simulink model "Model_DC_MG"  (R2024b)
settings: Solver=ode23tb  StartTime=0.0  StopTime=3  MaxStep=1e-2  RelTol=1e-3
InitFcn:
  | Main_DC_MG
undefined symbols (not defined in the file or in its folder): DiscIntNeverNeededParam, Ion, Lithium, R_Load_DC, sigbuilder_block, Ts_Control, Ts_Power, V2G, Vnom_DC
libraries: spsSeriesRLCBranchLib x9, spsMeanLib x9, simulink x8, spsBreakerLib x7, spsCurrentMeasurementLib x5, spsVoltageMeasurementLib x4, spsIGBTDiodeLib x2, spsFourierLib x2, spsPVArrayLib x1, spsBatteryLib x1, spsDiodeLib x1, spsIGBTLib x1
settings Model: Creator=Leony  LastModifiedBy=ASUS
settings SolverCC: ZeroCrossAlgorithm=Adaptive  AlgebraicLoopSolver=TrustRegion  SolverResetMethod=Robust
settings DataIOCC: LimitDataPoints=on  SaveFormat=Array  ReturnWorkspaceOutputs=off
settings OptimizationCC: LifeSpan=inf
settings DebuggingCC: AlgebraicLoopMsg=none  UnderspecifiedInitializationDetection=Classic  MergeDetectMultiDrivingBlocksExec=none  IgnoredZcDiagnostic=none  SolverPrmCheckMsg=warning  UnconnectedInputMsg=warning  UnconnectedOutputMsg=warning  UnconnectedLineMsg=warning  AllowSymbolicDim=off  SFUnexpectedBacktrackingDiag=warning  SFNoUnconditionalDefaultTransitionDiag=warning  SFExecutionAtInitializationDiag=none  ArithmeticOperatorsInVariantConditions=warning
settings HardwareCC: ProdBitPerPointer=32  ProdBitPerSizeT=32  ProdBitPerPtrDiffT=32  ProdLargestAtomicFloat=None  ProdIntDivRoundTo=Undefined  ProdEndianess=Unspecified  ProdWordSize=32  ProdHWDeviceType=32-bit Generic
settings ModelReferenceCC: EnableRefExpFcnMdlSchedulingChecks=on  PropagateSignalLabelsOutOfModel=off
settings SFSimCC: SimUseLocalCustomCode=off  CustomCodeUndefinedFunction=UseInterfaceOnly
settings RTWCC: RTWUseLocalCustomCode=off  GPUComputeCapability=3.5
settings CodeAppCC: StateflowObjectComments=on
settings GRTTargetCC: TargetLangStandard=C89/C90 (ANSI)
settings ConfigComp: CovMetricSettings=dw  CovSaveCumulativeToWorkspaceVar=on  CovSaveSingleToWorkspaceVar=on  CovExternalEMLEnable=off
settings SimscapeCC: SimscapeNormalizeSystem=off

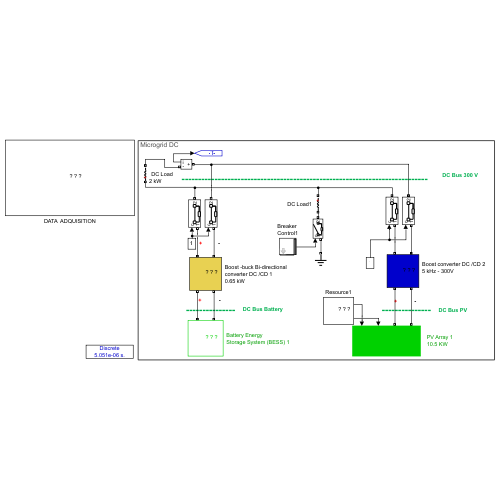
[thumbnail: Simulink's stored preview of the top-level diagram]
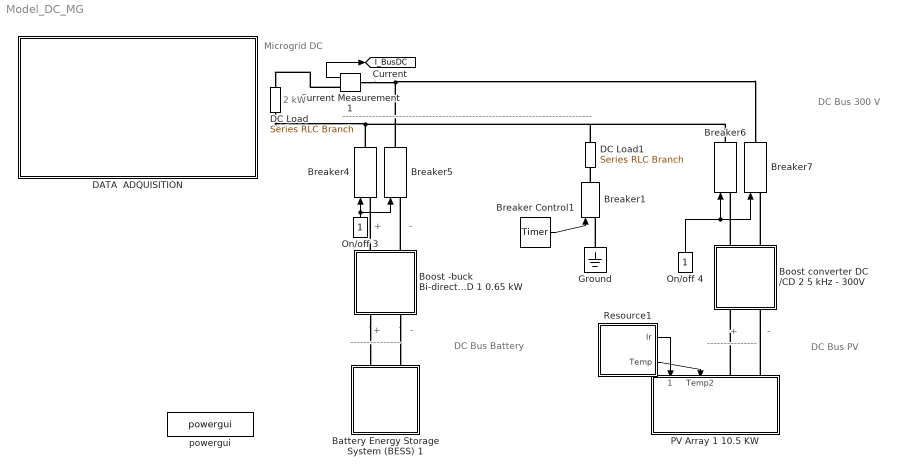
== system Model_DC_MG ==
  note: ---------------------------------------------------------------------------
  note: DC Bus 300 V
  note: 2 kW
  note: DC Bus Battery
  note: +
  note: -
  note: +
  note: ---------------
  note: -
  note: ---------------
  note: +
  note: -
  note: DC Bus PV
  note: Microgrid DC
  "  PV Array 1 10.5 KW" : Subsystem
      mask Display: image(imread('Icons\PV.png'));
  Battery Energy Storage System (BESS) 1 : Subsystem
      mask Display: image('Icons\Battery Energy Storage System (BESS).png');
  Boost -buck Bi-directional converter DC /CD 1 0.65 kW : Subsystem
      mask Display: image(imread('Icons\DC_DC_Converter.jpg'));
  "Boost converter DC /CD 2 5 kHz - 300V " : Subsystem
      mask Display: image(imread('Icons\DC_DC_Converter.jpg'));
  Breaker Control1 : powerlib_extras/Control  Blocks/Timer  t=[0 2 2.2]  e=[0 1 0]
  Breaker1 : spsBreakerLib/Breaker  InitialState=0  SwitchingTimes="[1/60  5/60]"  External=on  BreakerResistance=0.01  SnubberResistance=1e6  SnubberCapacitance=inf  Measurements=None  MoreParameters=on  NoBreakLoop=off
  Breaker{4..7} (4 alike) : spsBreakerLib/Breaker  InitialState=1  SwitchingTimes="[1/60  5/60]"  External=on  BreakerResistance=0.01  SnubberResistance=1e6  SnubberCapacitance=inf  Measurements=None  MoreParameters=on  NoBreakLoop=off
  Current Measurement1 : spsCurrentMeasurementLib/Current Measurement  PhasorSimulation=off  OutputType=Complex  PSBequivalent=0
  DATA  ADQUISITION : Subsystem
      mask Display: image('Icons\SCADA.png');
  DC Load : spsSeriesRLCBranchLib/Series RLC Branch  LConnTagsString=__new0  RConnTagsString=__new0  BranchType=R  Resistance=R_Load_DC  Inductance=1e-3  SetiL0=off  InitialCurrent=0  Capacitance=1e-6  Setx0=off  InitialVoltage=0  Measurements=None
  DC Load1 : spsSeriesRLCBranchLib/Series RLC Branch  LConnTagsString=__new0  RConnTagsString=__new0  BranchType=R  Resistance=0.001  Inductance=1e-3  SetiL0=off  InitialCurrent=0  Capacitance=1e-6  Setx0=off  InitialVoltage=0  Measurements=None
  Ground : spsGroundLib/Ground  LConnTagsString=a
  On/off 3 : Constant
  On/off 4 : Constant
  Resource1 : Subsystem
      mask Display: image(imread('Icons\R_Sol.jpg'));
  powergui : spspowerguiLib/powergui  Priority=1  SimulationMode=Discrete  SampleTime=Ts_Power  frequency=60  Iterations=50  frequencyindice=0  Pbase=100e6  ErrMax=1e-4  UnitsV=kV  UnitsW=MW  buscounter=0  FunctionMessages=off  echomessages=off  EnableUseOfTLC=off  CurrentSourceSwitches=off  DisableSnubberDevices=off  DisableRonSwitches=off  DisableVfSwitches=off  DisplayEquations=off  AutomaticDiscreteSolvers=off  SolverType=Tustin  Interpol=off  ExternalGateDelay=off  methode=off  Ts=0  x0status=blocks  SPID=off  SwTol=0  HookPort=off  NonlinearTolerance=1e-4  nMaxIteration=100  ContinueOnMaxIteration=off  RestoreLinks=warning  ResistiveCurrentMeasurement=off  Frange=[0:2:500]  Ylog=off  Xlog=on  ShowGrid=off  save=off  variable=ZData  structure=0  ZoomFFT=off  StartTime=0.0  cycles=1  DisplayStyle=1  fundamental=60  FreqAxis=off  MaxFrequency=1000  frequencyindicesteady=1  RmsSteady=1  display=off
  tag scope: I_BusDC=global
  wires:
  On/off 3/1 -> Breaker5/1, Breaker4/1
  Resource1/1(Ir) -> "  PV Array 1 10.5 KW"/1(Radiación)
  Resource1/2("Temp ") -> "  PV Array 1 10.5 KW"/2(Temp2)
  Current Measurement1/1 -> [I_BusDC]
  On/off 4/1 -> Breaker7/1, Breaker6/1
  Breaker Control1/1 -> Breaker1/1
  connections:
  Breaker5/RConn1 -- Current Measurement1/LConn1 -- Breaker7/RConn1
  Breaker4/RConn1 -- DC Load1/LConn1 -- Breaker6/RConn1 -- DC Load/LConn1
  Boost -buck Bi-directional converter DC /CD 1 0.65 kW/LConn1 -- Battery Energy Storage System (BESS) 1/LConn1
  Boost -buck Bi-directional converter DC /CD 1 0.65 kW/LConn2 -- Battery Energy Storage System (BESS) 1/LConn2
  Boost -buck Bi-directional converter DC /CD 1 0.65 kW/RConn1 -- Breaker4/LConn1
  Boost -buck Bi-directional converter DC /CD 1 0.65 kW/RConn2 -- Breaker5/LConn1
  "Boost converter DC /CD 2 5 kHz - 300V "/LConn1 -- Breaker6/LConn1
  "Boost converter DC /CD 2 5 kHz - 300V "/LConn2 -- Breaker7/LConn1
  "  PV Array 1 10.5 KW"/LConn2 -- "Boost converter DC /CD 2 5 kHz - 300V "/RConn2
  "  PV Array 1 10.5 KW"/LConn1 -- "Boost converter DC /CD 2 5 kHz - 300V "/RConn1
  Current Measurement1/RConn1 -- DC Load/RConn1
  Breaker1/RConn1 -- DC Load1/RConn1
  Ground/LConn1 -- Breaker1/LConn1

== system Model_DC_MG/  PV Array 1 10.5 KW ==
  note: DC Bus
  note: 10.5 - kW  PV Array
      | 42 * SunTech STP - 250S-20 /Wd  (Nser=6 Npar=7)
  Radiación : Inport
  Temp2 : Inport  Port=2
  PV Array : spsPVArrayLib/PV Array  Npar=7  Nser=6  PlotType=array @ 1000 W/m2 & specified temperatures  S_vec="[ 1000  250 ]"  Temp_C_vec="[0 25 50  ]"  ModuleName=User-defined  PlotWhenSelected=off  Pm=250.205  Ncell=96  Voc=37.4  Isc=8.63  Vm=30.7  Im=8.15  beta_Voc_pc=-0.34  alpha_Isc_pc=0.050  beta_Voc=-0.12716  alpha_Isc=0.004315  IL=8.6686  I0=1.3965e-10  nI=0.6105  Rsh=311.9016  Rs=0.26776  RobustModel=off  RobustCellTemperature=313.3991  BAL=on  Tc=Tc  Tfilter=5e-5
  + : PMIOPort  Tag=PMCPort  Side=Left
  - : PMIOPort  Tag=PMCPort  Port=2  Side=Left
  tag scope: m_PV=global
  wires:
  Temp2/1 -> PV Array/2
  Radiación/1 -> PV Array/1
  PV Array/1 -> [m_PV]
  connections:
  PV Array/RConn1 -- +/RConn1
  PV Array/RConn2 -- -/RConn1

== system Model_DC_MG/Battery Energy Storage System (BESS) 1 ==
  Battery1 : spsBatteryLib/Battery  BatType=Lithium-Ion  NomV=120  NomQ=800  SOC=80  Batt_Tr=3  PresetModel=on  MaxQ=800  MinV=90  FullV=139.6785  Dis_rate=347.8261  R=0.0015  Normal_OP=723.4783  expZone="[129.6463      39.30435]"
      settings: LibrarySourceBlock=electricdrivelib/Extra Sources/Battery
  + B1 : PMIOPort  Side=Left
  - B1 : PMIOPort  Port=2  Side=Left
  connections:
  Battery1/LConn2 -- - B1/RConn1
  Battery1/LConn1 -- + B1/RConn1

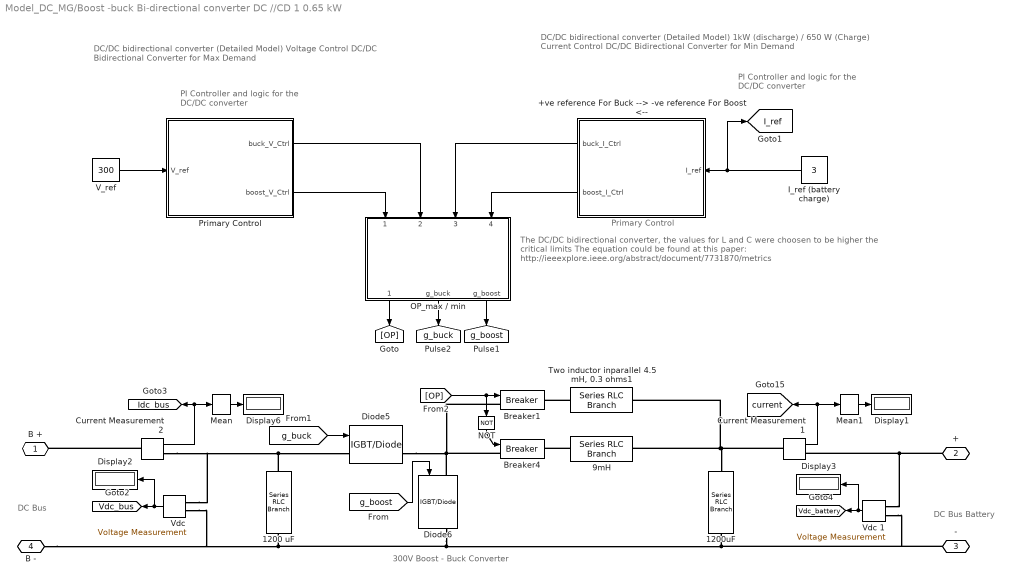
== system Model_DC_MG/Boost -buck Bi-directional converter DC //CD 1 0.65 kW ==
  note: Primary Control
  note: DC Bus
  note: DC Bus Battery
  note: PI Controller and logic for
      | the DC/DC converter
  note: DC/DC bidirectional converter (Detailed Model)
      | Voltage Control DC/DC Bidirectional Converter for Max Demand
  note: 300V
      | Boost - Buck Converter
  note: PI Controller and logic for
      | the DC/DC converter
  note: DC/DC bidirectional converter (Detailed Model)
      | 1kW (discharge) / 650 W (Charge)
      | Current Control DC/DC Bidirectional Converter for Min Demand
  note: The DC/DC bidirectional converter, the values for L and C were choosen to be higher the critical limits The equation could be found at this paper:
      | http://ieeexplore.ieee.org/abstract/document/7731870/metrics
  +ve reference For Buck --> -ve reference For Boost <-- : Subsystem
      mask Display: image('Icons\FPGA.png');
  1200 uF : spsSeriesRLCBranchLib/Series RLC Branch  LConnTagsString=__new0  RConnTagsString=__new0  BranchType=RC  Resistance=0.1  Inductance=3e-3  SetiL0=off  InitialCurrent=0  Capacitance=1200e-6  Setx0=off  InitialVoltage=150  Measurements=None
  1200uF : spsSeriesRLCBranchLib/Series RLC Branch  LConnTagsString=__new0  RConnTagsString=__new0  BranchType=C  Resistance=1  Inductance=3e-3  SetiL0=off  InitialCurrent=0  Capacitance=1200e-6  Setx0=off  InitialVoltage=130  Measurements=None
  9mH : spsSeriesRLCBranchLib/Series RLC Branch  LConnTagsString=__new0  RConnTagsString=__new0  BranchType=L  Resistance=1  Inductance=9e-3  SetiL0=off  InitialCurrent=0  Capacitance=1e-6  Setx0=off  InitialVoltage=0  Measurements=None
  Breaker1 : spsBreakerLib/Breaker  InitialState=0  SwitchingTimes="[1/60  5/60]"  External=on  BreakerResistance=0.0001  SnubberResistance=1e6  SnubberCapacitance=inf  Measurements=None  MoreParameters=on  NoBreakLoop=off
  Breaker4 : spsBreakerLib/Breaker  InitialState=0  SwitchingTimes="[1/60  5/60]"  External=on  BreakerResistance=0.0001  SnubberResistance=1e6  SnubberCapacitance=inf  Measurements=None  MoreParameters=on  NoBreakLoop=off
  Current Measurement1 : spsCurrentMeasurementLib/Current Measurement  PhasorSimulation=off  OutputType=Complex  PSBequivalent=0
  Current Measurement2 : spsCurrentMeasurementLib/Current Measurement  PhasorSimulation=off  OutputType=Complex  PSBequivalent=0
  Diode5 : spsIGBTDiodeLib/IGBT//Diode  Ron=1e-3  Rs=1e5  Cs=inf  Measurements=on
  Diode6 : spsIGBTDiodeLib/IGBT//Diode  Ron=1e-3  Rs=1e5  Cs=inf  Measurements=on
  Display{1..3,6} (4 alike) : Display
  I_ref (battery charge) : Constant  Value=3
  Mean : spsMeanLib/Mean  Freq=10  Vinit=0  Ts=0
  Mean1 : spsMeanLib/Mean  Freq=10  Vinit=0  Ts=0
  NOT : Logic  Operator=NOT  IconShape=distinctive  AllPortsSameDT=off  OutDataTypeStr=boolean
  OP_max / min : Subsystem
  Primary Control : Subsystem
      mask Display: image('Icons\FPGA.png');
  "Two inductor inparallel 4.5 mH, 0.3 ohms1" : spsSeriesRLCBranchLib/Series RLC Branch  LConnTagsString=__new0  RConnTagsString=__new0  BranchType=RL  Resistance=.25  Inductance=4.5e-3  SetiL0=off  InitialCurrent=0  Capacitance=1e-6  Setx0=off  InitialVoltage=0  Measurements=None
  V_ref : Constant  Value=300
  "Vdc " : spsVoltageMeasurementLib/Voltage Measurement  Tag=PoWeRsYsTeMmEaSuReMeNt  PhasorSimulation=off  OutputType=Magnitude  PSBequivalent=0
  Vdc 1 : spsVoltageMeasurementLib/Voltage Measurement  Tag=PoWeRsYsTeMmEaSuReMeNt  PhasorSimulation=off  OutputType=Magnitude  PSBequivalent=0
  B + : PMIOPort  Side=Right
  + : PMIOPort  Port=2  Side=Left
  - : PMIOPort  Port=3  Side=Left
  B - : PMIOPort  Port=4  Side=Right
  tag scope: I_ref=global, Idc_bus=global, Vdc_battery=global, Vdc_bus=global, current=global, g_boost=global, g_buck=global
  wires:
  "Vdc "/1 -> Display2/1, [Vdc_bus]
  Vdc 1/1 -> Display3/1, [Vdc_battery]
  Current Measurement2/1 -> Mean/1, [Idc_bus]
  [g_boost] -> Diode6/1
  [g_buck] -> Diode5/1
  Mean/1 -> Display6/1
  Current Measurement1/1 -> [current], Mean1/1
  Mean1/1 -> Display1/1
  V_ref/1 -> Primary Control/1(V_ref)
  OP_max / min/1(Op_Max / Min) -> [OP]
  [OP] -> NOT/1, Breaker1/1
  NOT/1 -> Breaker4/1
  I_ref (battery charge)/1 -> [I_ref], +ve reference For Buck --> -ve reference For Boost <--/1(I_ref)
  +ve reference For Buck --> -ve reference For Boost <--/1(buck_I_Ctrl) -> OP_max / min/3(buck_I_Ctrl)
  +ve reference For Buck --> -ve reference For Boost <--/2(boost_I_Ctrl) -> OP_max / min/4(boost_I_Ctrll)
  OP_max / min/2(g_buck) -> [g_buck]
  OP_max / min/3(g_boost) -> [g_boost]
  Primary Control/1(buck_V_Ctrl) -> OP_max / min/2(buck_V_Ctrl)
  Primary Control/2(boost_V_Ctrl) -> OP_max / min/1(boost_V_Ctrll)
  connections:
  +/RConn1 -- Vdc 1/LConn1 -- Current Measurement1/RConn1
  Diode5/RConn1 -- Breaker1/LConn1 -- Breaker4/LConn1 -- Diode6/LConn1
  1200 uF/LConn1 -- "Vdc "/LConn1 -- Current Measurement2/RConn1 -- Diode5/LConn1
  Diode6/RConn1 -- "Vdc "/LConn2 -- B -/RConn1 -- 1200 uF/RConn1 -- Vdc 1/LConn2 -- -/RConn1 -- 1200uF/RConn1
  Current Measurement2/LConn1 -- B +/RConn1
  "Two inductor inparallel 4.5 mH, 0.3 ohms1"/LConn1 -- Breaker1/RConn1
  Current Measurement1/LConn1 -- 1200uF/LConn1 -- 9mH/RConn1 -- "Two inductor inparallel 4.5 mH, 0.3 ohms1"/RConn1
  9mH/LConn1 -- Breaker4/RConn1

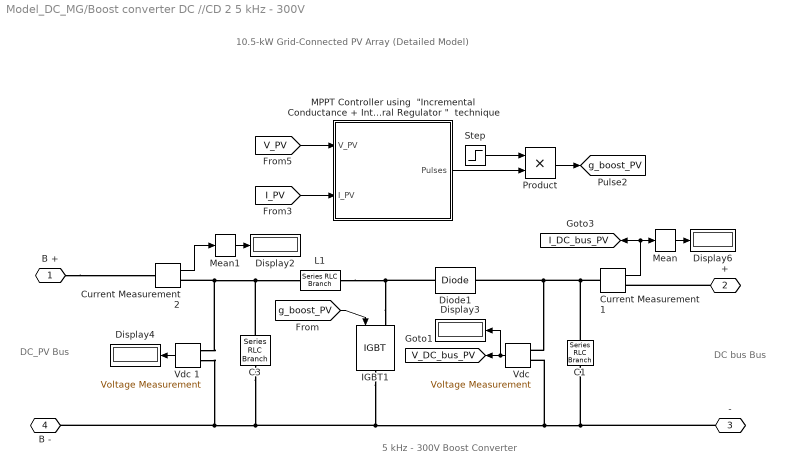
== system Model_DC_MG/Boost converter DC //CD 2 5 kHz - 300V  ==
  note: DC_PV Bus
  note: DC bus Bus
  note: 5 kHz - 300V
      | Boost Converter
  note: 10.5-kW Grid-Connected PV Array (Detailed Model)
  C1 : spsSeriesRLCBranchLib/Series RLC Branch  LConnTagsString=__new0  RConnTagsString=__new0  BranchType=C  Resistance=1.0  Inductance=1.0  SetiL0=off  InitialCurrent=0  Capacitance=6000e-06  Setx0=off  InitialVoltage=0  Measurements=None
  C3 : spsSeriesRLCBranchLib/Series RLC Branch  LConnTagsString=__new0  RConnTagsString=__new0  BranchType=C  Resistance=1.0  Inductance=1.0  SetiL0=off  InitialCurrent=0  Capacitance=100e-6  Setx0=off  InitialVoltage=0  Measurements=Branch voltage
  Current Measurement1 : spsCurrentMeasurementLib/Current Measurement  PhasorSimulation=off  OutputType=Complex  PSBequivalent=0
  Current Measurement2 : spsCurrentMeasurementLib/Current Measurement  PhasorSimulation=off  OutputType=Complex  PSBequivalent=0
  Diode1 : spsDiodeLib/Diode  Ron=1e-4  Lon=0  Vf=0  IC=0  UseSnubber=off  Rs=inf  Cs=inf  Measurements=off
  Display{2..4,6} (4 alike) : Display
  IGBT1 : spsIGBTLib/IGBT  Ron=0.001  Lon=0  Vf=0  Tf=0  Tt=0  IC=0  Rs=1e5  Cs=inf  Measurements=off
  L1 : spsSeriesRLCBranchLib/Series RLC Branch  LConnTagsString=__new0  RConnTagsString=__new0  BranchType=RL  Resistance=0.005  Inductance=5e-3  SetiL0=off  InitialCurrent=0  Capacitance=1e-6  Setx0=off  InitialVoltage=0  Measurements=None
  "MPPT Controller using  \"Incremental Conductance + Integral Regulator \"  technique " : Subsystem  mask(Boost Control - MPPT){fc=5000, T_MPPT=200e-6, Dinit=0.25}
      mask prompts: fc "PWM switching frequency (Hz)"; T_MPPT "Time window used by MPPT control (s)"; Dinit "Initial value of duty cycle"
      mask Display: image('Icons\FPGA.png');
  Mean : spsMeanLib/Mean  Freq=10  Vinit=0  Ts=0
  Mean1 : spsMeanLib/Mean  Freq=10  Vinit=0  Ts=0
  Product : Product
  Step : Step  Time=0  SampleTime=0
  "Vdc " : spsVoltageMeasurementLib/Voltage Measurement  Tag=PoWeRsYsTeMmEaSuReMeNt  PhasorSimulation=off  OutputType=Magnitude  PSBequivalent=0
  Vdc 1 : spsVoltageMeasurementLib/Voltage Measurement  Tag=PoWeRsYsTeMmEaSuReMeNt  PhasorSimulation=off  OutputType=Magnitude  PSBequivalent=0
  B + : PMIOPort  Side=Right
  + : PMIOPort  Port=2  Side=Left
  - : PMIOPort  Port=3  Side=Left
  B - : PMIOPort  Port=4  Side=Right
  tag scope: I_DC_bus_PV=global, V_DC_bus_PV=global, g_boost_PV=global
  wires:
  [I_PV] -> "MPPT Controller using  \"Incremental Conductance + Integral Regulator \"  technique "/2(I_PV)
  "MPPT Controller using  \"Incremental Conductance + Integral Regulator \"  technique "/1(Pulses) -> Product/2
  [V_PV] -> "MPPT Controller using  \"Incremental Conductance + Integral Regulator \"  technique "/1(V_PV)
  Step/1 -> Product/1
  Current Measurement2/1 -> Mean1/1
  Mean/1 -> Display6/1
  Current Measurement1/1 -> [I_DC_bus_PV], Mean/1
  "Vdc "/1 -> Display3/1, [V_DC_bus_PV]
  Product/1 -> [g_boost_PV]
  [g_boost_PV] -> IGBT1/1
  Vdc 1/1 -> Display4/1
  Mean1/1 -> Display2/1
  connections:
  Current Measurement2/RConn1 -- Vdc 1/LConn1 -- L1/LConn1 -- C3/LConn1
  C3/RConn1 -- -/RConn1 -- C1/RConn1 -- "Vdc "/LConn2 -- IGBT1/RConn1 -- B -/RConn1 -- Vdc 1/LConn2
  IGBT1/LConn1 -- Diode1/LConn1 -- L1/RConn1
  B +/RConn1 -- Current Measurement2/LConn1
  +/RConn1 -- Current Measurement1/RConn1
  C1/LConn1 -- Current Measurement1/LConn1 -- Diode1/RConn1 -- "Vdc "/LConn1

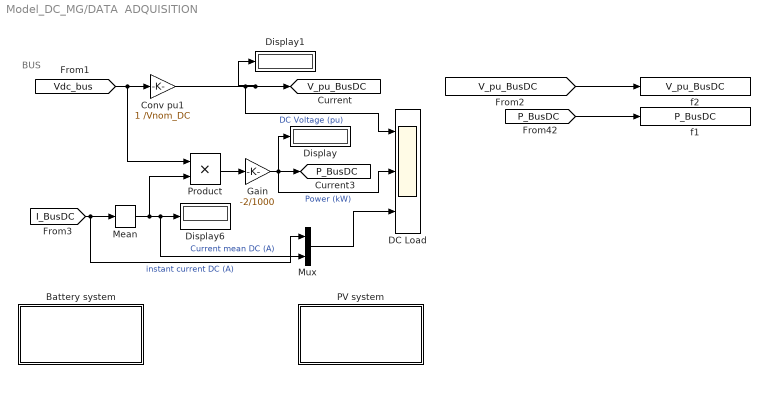
== system Model_DC_MG/DATA  ADQUISITION ==
  note: BUS
  Battery system : Subsystem
      mask Display: disp('Open this block\nto display additional \nscopes & measurements')
  Conv pu1 : Gain  Gain=1 /Vnom_DC  SaturateOnIntegerOverflow=on  OutDataTypeStr=Inherit: Same as input  ParamDataTypeStr=Inherit: Same as input
  DC Load : Scope  NumInputPorts=3
  Display : Display
  Display1 : Display
  Display6 : Display
  Gain : Gain  Gain=-2/1000
  Mean : spsMeanLib/Mean  Freq=10  Vinit=0  Ts=0
  Mux : Mux  Inputs=2
  PV system : Subsystem
      mask Display: disp('Open this block\nto display additional \nscopes & measurements')
  Product : Product
  f1 : ToWorkspace  VariableName=P_BusDC  SaveFormat=Timeseries  SampleTime=-1
  f2 : ToWorkspace  VariableName=V_pu_BusDC  SaveFormat=Timeseries  SampleTime=-1
  tag scope: P_BusDC=global, V_pu_BusDC=global
  wires:
  [V_pu_BusDC] -> f2/1
  [P_BusDC] -> f1/1
  Gain/1 -> Display/1, DC Load/2, [P_BusDC]  "Power (kW)"
  Product/1 -> Gain/1
  Mux/1 -> DC Load/3
  Mean/1 -> Product/2, Mux/2, Display6/1  "Current mean DC (A)"
  [I_BusDC] -> Mux/1, Mean/1  "instant current DC (A)"
  [Vdc_bus] -> Product/1, Conv pu1/1
  Conv pu1/1 -> DC Load/1, Display1/1, [V_pu_BusDC]  "DC Voltage (pu)"

== system Model_DC_MG/Resource1 ==
  Irradiance : Subsystem  Commented=on
      mask init:
      | load power_V2G
      mask Display: plot(V2G.IRRADIANCE.time,V2G.IRRADIANCE.SUN)
  Irradiance (W/m^2) : Display
      settings: Format=bank  Decimation=1000
  Irradiance Temp Demand Max : Subsystem  Tag=STV Subsys  LoadFcn=sigbuilder_block('load');  StartFcn=sigbuilder_block('start');  StopFcn=sigbuilder_block('stop');  ClipboardFcn=sigbuilder_block('clipboard');  mask(Sigbuilder block){tuvar=[0:10]}
      mask help: Sigbuilder GUI
      mask init:
      | if ~strcmp(get_param(bdroot(gcbh),'SimulationStatus'),'stopped') tuvar = sigbuilder_block('maskInit'); end
      settings: CopyFcn=sigbuilder_block('copy');  DeleteFcn=sigbuilder_block('delete');  ModelCloseFcn=sigbuilder_block('modelClose');  PreSaveFcn=sigbuilder_block('preSave');  PauseFcn=sigbuilder_block('pause')  ContinueFcn=sigbuilder_block('continue')  NameChangeFcn=sigbuilder_block('namechange');  OpenFcn=sigbuilder_block('open',[5.4 30 1141.2 522.6 ]);  CloseFcn=sigbuilder_block('close');
      mask Display: plot(0, 0, 100, 100,[2, 2, 32, 32, 2], [68, 8, 8, 68, 68],[32, 2], [38, 38], [32, 19, 2],[53, 60, 44], [32, 17, 17, 2],[16, 16, 31, 31]);txt = getActiveGroup(gcbh);text(2, 100, txt,'verticalAlignment', 'top');
  Partial Shading : Subsystem  Commented=on  mask(Signal Disturbance){Hour=0, Minute=0, Second=1, Duration=1/44, Factor=0.7}
      mask prompts: Duration "Duration (s):"
      mask help: Within the specified time range defined by Start and Duration parameters, output is set to 'Factor'. Outside the specified time range output is kept at 1.0.
      mask init:
      | T2=(Hour-1)*60*60;    % Hour in seconds
      | T3=(Minute-1)*60;  % Minute in seconds
      | Ton=T2+T3+(Second-1);    % Beginning of fault (s)
      | Toff=Ton+Duration; % End of fault (s)
      mask TypeOptions Hour: 0 |      1 |      2 |      3 |      4 |      5 |      6 |      7 |      8 |      9 |     10 |     11 |     12 |     13 |     14 |     15 |     16 |     17 |     18 |     19 |     20 |     21 |     22 |     23
      mask TypeOptions Minute: 0 |      1 |      2 |      3 |      4 |      5 |      6 |      7 |      8 |      9 |     10 |     11 |     12 |     13 |     14 |     15 |     16 |     17 |     18 |     19 |     20 |     21 |     22 |     23 |     24 |     25 |     26 |     27 |     28 |     29 |     30 |     31 |     32 |     33 |     34 |     35 |     36 |     37 |     38 |     39 |     40 |     41 |     42 |     43 |     44 |     45 |     46 |     47 |     48 |     49 |     50 |     51 |     52 |     53 |     54 |     55 |     56 |     57 |     58 |     59
      mask TypeOptions Second: 0 |      1 |      2 |      3 |      4 |      5 |      6 |      7 |      8 |      9 |     10 |     11 |     12 |     13 |     14 |     15 |     16 |     17 |     18 |     19 |     20 |     21 |     22 |     23 |     24 |     25 |     26 |     27 |     28 |     29 |     30 |     31 |     32 |     33 |     34 |     35 |     36 |     37 |     38 |     39 |     40 |     41 |     42 |     43 |     44 |     45 |     46 |     47 |     48 |     49 |     50 |     51 |     52 |     53 |     54 |     55 |     56 |     57 |     58 |     59
      mask DialogControl Control2 Prompt: Start:
  Product1 : Product  Commented=on
  Rate Limiter2 : RateLimiter  Commented=on  RisingSlewLimit=1e4  FallingSlewLimit=-1e4  SampleTimeMode=inherited
  Temperature (deg. C) : Display
      settings: Format=bank  Decimation=1000
  Ir : Outport  VectorParamsAs1DForOutWhenUnconnected=off
  "Temp " : Outport  Port=2  VectorParamsAs1DForOutWhenUnconnected=off
  wires:
  Irradiance/1(" ") -> Product1/1
  Partial Shading/1(Out) -> Product1/2
  Product1/1 -> Rate Limiter2/1
  Irradiance Temp Demand Max/1(Ir) -> Irradiance (W/m^2)/1, Ir/1
  Irradiance Temp Demand Max/2(Temp) -> Temperature (deg. C)/1, "Temp "/1

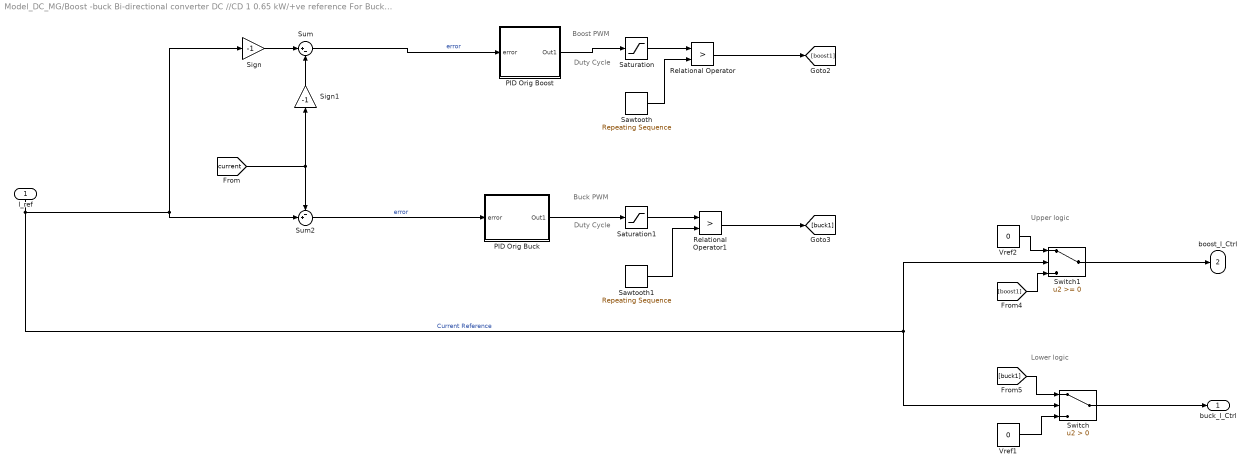
== system Model_DC_MG/Boost -buck Bi-directional converter DC //CD 1 0.65 kW/+ve reference For Buck --> -ve reference For Boost <-- ==
  note: Buck PWM
  note: Duty Cycle
  note: Upper logic
  note: Lower logic
  note: Boost PWM
  note: Duty Cycle
  I_ref : Inport
  PID Orig Boost : Subsystem
  PID Orig Buck : Subsystem
  Relational Operator : RelationalOperator  Operator=>  OutDataTypeStr=boolean  InputSameDT=off
  Relational Operator1 : RelationalOperator  Operator=>  OutDataTypeStr=boolean  InputSameDT=off
  Saturation : Saturate  UpperLimit=0.9  LowerLimit=0
  Saturation1 : Saturate  UpperLimit=0.8  LowerLimit=0
  Sawtooth : simulink/Sources/Repeating Sequence  rep_seq_t=[0 1/5000]  rep_seq_y=[0 1]
  Sawtooth1 : simulink/Sources/Repeating Sequence  rep_seq_t=[0 1/5000]  rep_seq_y=[0 1]
  Sign : Gain  Gain=-1
  Sign1 : Gain  Gain=-1
  Sum : Sum  Inputs=|+-
  Sum2 : Sum  Inputs=-+|
  Switch : Switch  Criteria=u2 > Threshold  SaturateOnIntegerOverflow=off  InputSameDT=off
  Switch1 : Switch  SaturateOnIntegerOverflow=off  InputSameDT=off
  Vref1 : Constant  Value=0
  Vref2 : Constant  Value=0
  buck_I_Ctrl : Outport  VectorParamsAs1DForOutWhenUnconnected=off
  boost_I_Ctrl : Outport  Port=2  VectorParamsAs1DForOutWhenUnconnected=off
  wires:
  Sum/1 -> PID Orig Boost/1(error)  "error"
  Relational Operator/1 -> [boost1]
  Sign/1 -> Sum/1
  PID Orig Boost/1(Out1) -> Saturation/1
  PID Orig Buck/1(Out1) -> Saturation1/1
  Sawtooth/1 -> Relational Operator/2
  Sawtooth1/1 -> Relational Operator1/2
  Relational Operator1/1 -> [buck1]
  Sum2/1 -> PID Orig Buck/1(error)  "error"
  Saturation/1 -> Relational Operator/1
  Saturation1/1 -> Relational Operator1/1
  Vref1/1 -> Switch/3
  Vref2/1 -> Switch1/1
  [boost1] -> Switch1/3
  [buck1] -> Switch/1
  I_ref/1 -> Switch1/2, Switch/2, Sum2/2, Sign/1  "Current Reference"
  Sign1/1 -> Sum/2
  Switch1/1 -> boost_I_Ctrl/1
  Switch/1 -> buck_I_Ctrl/1
  [current] -> Sum2/1, Sign1/1

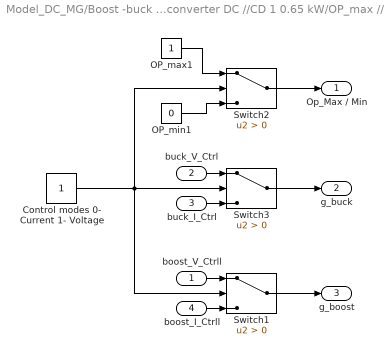
== system Model_DC_MG/Boost -buck Bi-directional converter DC //CD 1 0.65 kW/OP_max // min ==
  boost_V_Ctrll : Inport
  buck_V_Ctrl : Inport  Port=2
  buck_I_Ctrl : Inport  Port=3
  boost_I_Ctrll : Inport  Port=4
  Control modes 0- Current 1- Voltage : Constant
  OP_max1 : Constant
  OP_min1 : Constant  Value=0
  Switch1 : Switch  Criteria=u2 > Threshold  SaturateOnIntegerOverflow=off  InputSameDT=off
  Switch2 : Switch  Criteria=u2 > Threshold  SaturateOnIntegerOverflow=off  InputSameDT=off
  Switch3 : Switch  Criteria=u2 > Threshold  SaturateOnIntegerOverflow=off  InputSameDT=off
  Op_Max / Min : Outport  VectorParamsAs1DForOutWhenUnconnected=off
  g_buck : Outport  Port=2  VectorParamsAs1DForOutWhenUnconnected=off
  g_boost : Outport  Port=3  VectorParamsAs1DForOutWhenUnconnected=off
  wires:
  OP_max1/1 -> Switch2/1
  OP_min1/1 -> Switch2/3
  Switch2/1 -> Op_Max / Min/1
  Control modes 0- Current 1- Voltage/1 -> Switch2/2, Switch1/2, Switch3/2
  boost_I_Ctrll/1 -> Switch1/3
  boost_V_Ctrll/1 -> Switch1/1
  buck_V_Ctrl/1 -> Switch3/1
  buck_I_Ctrl/1 -> Switch3/3
  Switch1/1 -> g_boost/1
  Switch3/1 -> g_buck/1

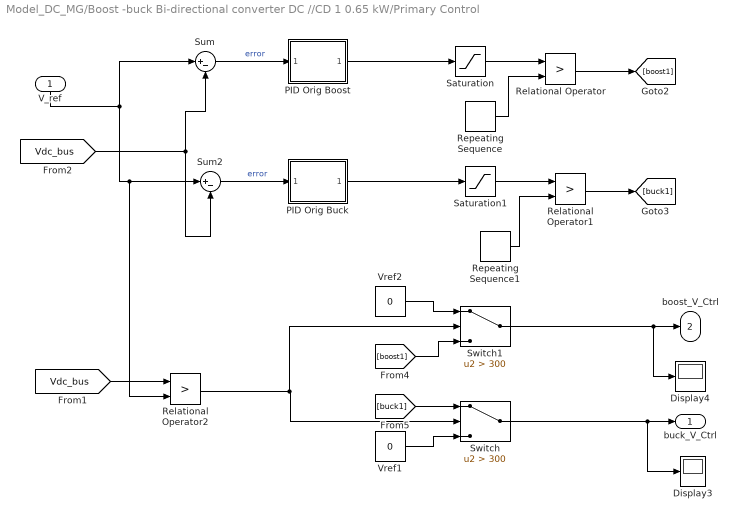
== system Model_DC_MG/Boost -buck Bi-directional converter DC //CD 1 0.65 kW/Primary Control ==
  V_ref : Inport
  Display3 : Display
  Display4 : Display
  PID Orig Boost : Subsystem
  PID Orig Buck : Subsystem
  Relational Operator : RelationalOperator  Operator=>  OutDataTypeStr=boolean  InputSameDT=off
  Relational Operator1 : RelationalOperator  Operator=>  OutDataTypeStr=boolean  InputSameDT=off
  Relational Operator2 : RelationalOperator  Operator=>  OutDataTypeStr=boolean  InputSameDT=off
  Repeating Sequence : simulink/Sources/Repeating Sequence  rep_seq_t=[0 1/5000]  rep_seq_y=[0 1]
  Repeating Sequence1 : simulink/Sources/Repeating Sequence  rep_seq_t=[0 1/5000]  rep_seq_y=[0 1]
  Saturation : Saturate  UpperLimit=0.9  LowerLimit=0
  Saturation1 : Saturate  UpperLimit=0.9  LowerLimit=0
  Sum : Sum  Inputs=|+-
  Sum2 : Sum  Inputs=|+-
  Switch : Switch  Criteria=u2 > Threshold  Threshold=300  SaturateOnIntegerOverflow=off  InputSameDT=off
  Switch1 : Switch  Criteria=u2 > Threshold  Threshold=300  SaturateOnIntegerOverflow=off  InputSameDT=off
  Vref1 : Constant  Value=0
  Vref2 : Constant  Value=0
  buck_V_Ctrl : Outport  VectorParamsAs1DForOutWhenUnconnected=off
  boost_V_Ctrl : Outport  Port=2  VectorParamsAs1DForOutWhenUnconnected=off
  wires:
  Relational Operator2/1 -> Switch1/2, Switch/2
  Saturation1/1 -> Relational Operator1/1
  V_ref/1 -> Sum/1, Relational Operator2/2, Sum2/1
  [Vdc_bus] -> Relational Operator2/1
  Vref2/1 -> Switch1/1
  Repeating Sequence/1 -> Relational Operator/2
  Repeating Sequence1/1 -> Relational Operator1/2
  Relational Operator1/1 -> [buck1]
  [Vdc_bus] -> Sum2/2, Sum/2
  [buck1] -> Switch/1
  Switch1/1 -> Display4/1, boost_V_Ctrl/1
  Saturation/1 -> Relational Operator/1
  [boost1] -> Switch1/3
  Sum2/1 -> PID Orig Buck/1(error)  "error"
  Relational Operator/1 -> [boost1]
  Switch/1 -> Display3/1, buck_V_Ctrl/1
  Vref1/1 -> Switch/3
  Sum/1 -> PID Orig Boost/1(error)  "error"
  PID Orig Buck/1(Out1) -> Saturation1/1
  PID Orig Boost/1(Out1) -> Saturation/1

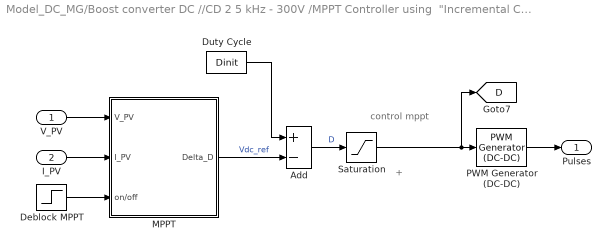
== system Model_DC_MG/Boost converter DC //CD 2 5 kHz - 300V /MPPT Controller using  "Incremental Conductance + Integral Regulator "  technique  ==
  note: +
  note: control mppt
  V_PV : Inport
  I_PV : Inport  Port=2
  Add : Sum  Inputs=+-
  Deblock MPPT : Step  Time=0.2  SampleTime=0
  Duty Cycle : Constant  Value=Dinit
  MPPT : Subsystem
  PWM Generator (DC-DC) : spsPWMGeneratorDCDCLib/PWM Generator (DC-DC)  Fsw=fc  Ts=Ts_Power
  Saturation : Saturate  UpperLimit=1  LowerLimit=0
  Pulses : Outport  VectorParamsAs1DForOutWhenUnconnected=off
  tag scope: D=global
  wires:
  V_PV/1 -> MPPT/1(V_PV)
  I_PV/1 -> MPPT/2(I_PV)
  PWM Generator (DC-DC)/1 -> Pulses/1
  Deblock MPPT/1 -> MPPT/3(on/off)
  Add/1 -> Saturation/1  "D"
  MPPT/1(Delta_D) -> Add/2  "Vdc_ref"
  Duty Cycle/1 -> Add/1
  Saturation/1 -> [D], PWM Generator (DC-DC)/1

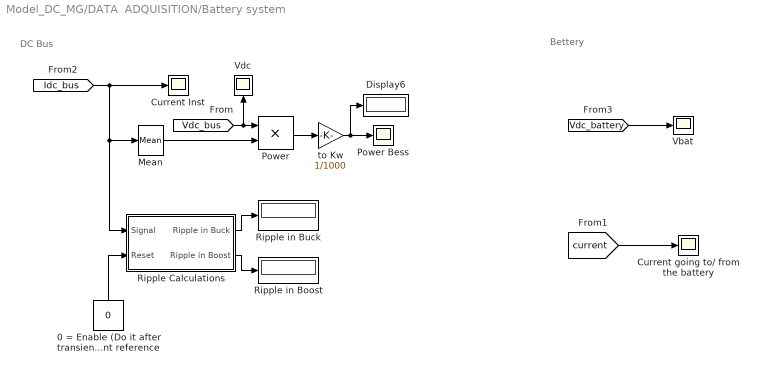
== system Model_DC_MG/DATA  ADQUISITION/Battery system ==
  note: DC Bus
  note: Bettery
  "0 = Enable (Do it after transient, so that it does not calculate ripples during transient) 1 = Reset after every change in current reference" : Constant  Value=0
  Current Inst : Scope
  Current going to/ from the battery : Scope
  Display6 : Display
  Mean : spsMeanLib/Mean  Freq=10  Vinit=0  Ts=0
  Power : Product
  Power Bess : Scope
  Ripple Calculations : Subsystem
  Ripple in Boost : Display
  Ripple in Buck : Display
  Vbat : Scope
  Vdc : Scope
  to Kw : Gain  Gain=1/1000
  wires:
  to Kw/1 -> Display6/1, Power Bess/1
  Mean/1 -> Power/2
  Power/1 -> to Kw/1
  Ripple Calculations/1(Ripple in Buck) -> Ripple in Buck/1
  "0 = Enable (Do it after transient, so that it does not calculate ripples during transient) 1 = Reset after every change in current reference"/1 -> Ripple Calculations/2(Reset)
  Ripple Calculations/2(Ripple in Boost) -> Ripple in Boost/1
  [Idc_bus] -> Mean/1, Ripple Calculations/1(Signal), Current Inst/1
  [current] -> Current going to/ from the battery/1
  [Vdc_bus] -> Vdc/1, Power/1
  [Vdc_battery] -> Vbat/1

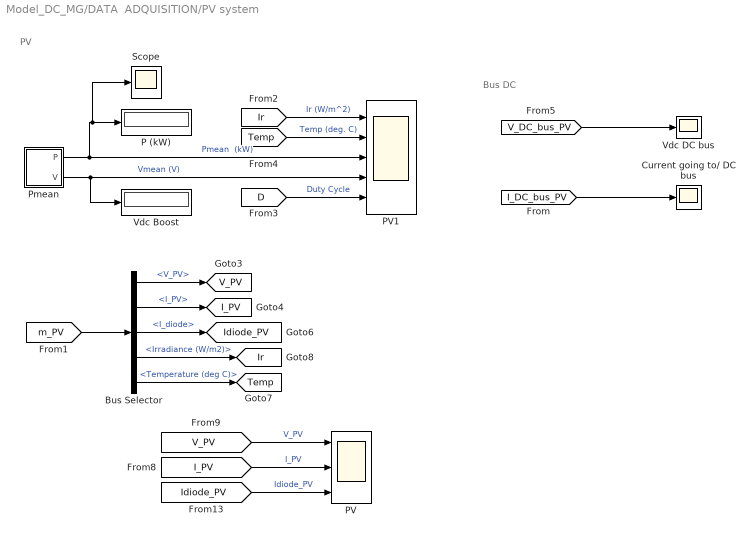
== system Model_DC_MG/DATA  ADQUISITION/PV system ==
  note: Bus DC
  note: PV
  Bus Selector : BusSelector  OutputSignals=V_PV,I_PV,I_diode,Irradiance (W/m2),Temperature (deg C)
  Current going to/ DC bus : Scope
  "P (kW) " : Display
      settings: Format=bank  Decimation=2000
  PV : Scope  NumInputPorts=3
  PV1 : Scope  NumInputPorts=5
  Pmean : Subsystem
  Scope : Scope
  Vdc Boost : Display
      settings: Format=bank  Decimation=2000
  Vdc DC bus : Scope
  tag scope: I_PV=global, Idiode_PV=global, Ir=global, Temp=global, V_PV=global
  wires:
  [V_PV] -> PV/1  "V_PV"
  [I_PV] -> PV/2  "I_PV"
  [Idiode_PV] -> PV/3  "Idiode_PV"
  [m_PV] -> Bus Selector/1
  Bus Selector/1 -> [V_PV]  "<V_PV>"
  Bus Selector/2 -> [I_PV]  "<I_PV>"
  Bus Selector/4 -> [Ir]  "<Irradiance (W/m2)>"
  Bus Selector/3 -> [Idiode_PV]  "<I_diode>"
  Bus Selector/5 -> [Temp]  "<Temperature (deg C)>"
  [Temp] -> PV1/2  "Temp (deg. C)"
  [D] -> PV1/5  "Duty Cycle"
  Pmean/2(V) -> Vdc Boost/1, PV1/4  "Vmean (V)"
  [Ir] -> PV1/1  "Ir (W/m^2)"
  Pmean/1(P) -> Scope/1, "P (kW) "/1, PV1/3  "Pmean  (kW)"
  [I_DC_bus_PV] -> Current going to/ DC bus/1
  [V_DC_bus_PV] -> Vdc DC bus/1

== system Model_DC_MG/Resource1/Irradiance ==
  1-D Lookup IRRADIANCE Table : Lookup_n-D  NumberOfTableDimensions=1  BreakpointsForDimension1=V2G.IRRADIANCE.time  BeginIndexSearchUsingPreviousIndexResult=on  Table=V2G.IRRADIANCE.SUN  InternalRulePriority=Speed  RndMeth=Simplest
  Add : Sum
  Clock1 : Clock
  Constant1 : Constant
  Second-->Hour : Gain  Gain=24/2
  " " : Outport  VectorParamsAs1DForOutWhenUnconnected=off
  wires:
  Constant1/1 -> Add/2
  Add/1 -> 1-D Lookup IRRADIANCE Table/1  "Hour of the day"
  1-D Lookup IRRADIANCE Table/1 -> " "/1
  Clock1/1 -> Second-->Hour/1
  Second-->Hour/1 -> Add/1

== system Model_DC_MG/Resource1/Irradiance Temp Demand Max ==
  Demux : Demux  Tag=STV Demux  Outputs=2
      settings: DisplayOption=none
  FromWs : FromWorkspace  Tag=STV FromWs  VariableName=tuvar
      SigBuilderData=|
      | common.afterFinalStr = 'Extrapolate'
      | common.sampleTime = '0'
      | dataSet(1).timeRange = [0 2]
      | dataSet(1).name = 'Constant Irradiance'
      | dataSet(2).timeRange = [0 2]
      | dataSet(2).name = 'Step Irradiance'
      | dataSet(3).timeRange = [0 3]
      | dataSet(3).name = 'Ramp-up/down Irradiance'
      | sbobj.Groups(1).Name = 'Constant Irradiance'
      | sbobj.Groups(1).Signals(1).Name = 'Ir'
      | sbobj.Groups(1).Signals(1).XData = [0 2]
      | sbobj.Groups(1).Signals(1).YData = [1000 1000]
      | sbobj.Groups(1).Signals(2).Name = 'Temp'
      | sbobj.Groups(1).Signals(2).XData = [0 1 1 2]
      | sbobj.Groups(1).Signals(2).YData = [0 0 1 1]
      | sbobj.Groups(1).TimeRange = [0 2]
      | sbobj.Groups(2).Name = 'Step Irradiance'
      | sbobj.Groups(2).Signals(1).Name = 'Ir'
      | sbobj.Groups(2).Signals(1).XData = [0 0.252 0.252 2]
      | sbobj.Groups(2).Signals(1).YData = [600 600 1000 1000]
      | sbobj.Groups(2).Signals(2).Name = 'Temp'
      | sbobj.Groups(2).Signals(2).XData = [0 1 1 2]
      | sbobj.Groups(2).Signals(2).YData = [0 0 1 1]
      | sbobj.Groups(2).TimeRange = [0 2]
      | sbobj.Groups(3).Name = 'Ramp-up/down Irradiance'
      | sbobj.Groups(3).Signals(1).Name = 'Ir'
      | sbobj.Groups(3).Signals(1).XData = [0 0.175 0.185 0.2 0.235 0.25 0.25 0.315 0.33 0.355 0.44 3]
      | sbobj.Groups(3).Signals(1).YData = [1000.5 1000.12765957 977.5 1000.07446809 1000 986.5 1000 1000 992 1000 1000 1000]
      | sbobj.Groups(3).Signals(2).Name = 'Temp'
      | sbobj.Groups(3).Signals(2).XData = [0 3]
      | sbobj.Groups(3).Signals(2).YData = [25 25]
      | sbobj.Groups(3).TimeRange = [0 3]
  Ir : Outport  Tag=STV Outport  VectorParamsAs1DForOutWhenUnconnected=off
  Temp : Outport  Tag=STV Outport  Port=2  VectorParamsAs1DForOutWhenUnconnected=off
  wires:
  Demux/1 -> Ir/1
  FromWs/1 -> Demux/1
  Demux/2 -> Temp/1

== system Model_DC_MG/Resource1/Partial Shading ==
  Add : Sum
  Clock : Clock
  Compare To Constant : simulink/Logic and Bit Operations/Compare To Constant  relop=>=  const=Ton  OutDataTypeStr=boolean
  Compare To Constant1 : simulink/Logic and Bit Operations/Compare To Constant  relop=<  const=Toff  OutDataTypeStr=boolean
  Constant : Constant  Value=Factor
  Logical Operator : Logic  AllPortsSameDT=off  OutDataTypeStr=float('double')
  Logical Operator1 : Logic  Operator=NOT  AllPortsSameDT=off  OutDataTypeStr=float('double')
  Product : Product
  Out : Outport  VectorParamsAs1DForOutWhenUnconnected=off
  wires:
  Add/1 -> Out/1
  Product/1 -> Add/2
  Constant/1 -> Product/2
  Compare To Constant/1 -> Logical Operator/1
  Clock/1 -> Compare To Constant1/1, Compare To Constant/1
  Compare To Constant1/1 -> Logical Operator/2
  Logical Operator/1 -> Logical Operator1/1, Product/1
  Logical Operator1/1 -> Add/1

== system Model_DC_MG/Boost -buck Bi-directional converter DC //CD 1 0.65 kW/+ve reference For Buck --> -ve reference For Boost <--/PID Orig Boost ==
  error : Inport
  Integrator2 : Integrator  LimitOutput=on  UpperSaturationLimit=0.9  LowerSaturationLimit=0
  Ki2 : Gain  Gain=3
  Kp2 : Gain  Gain=0.02
  Sum4 : Sum  Inputs=|++
  Out1 : Outport  VectorParamsAs1DForOutWhenUnconnected=off
  wires:
  error/1 -> Kp2/1, Ki2/1
  Kp2/1 -> Sum4/1
  Sum4/1 -> Out1/1
  Ki2/1 -> Integrator2/1
  Integrator2/1 -> Sum4/2

== system Model_DC_MG/Boost -buck Bi-directional converter DC //CD 1 0.65 kW/+ve reference For Buck --> -ve reference For Boost <--/PID Orig Buck ==
  error : Inport
  Integrator3 : Integrator  LimitOutput=on  UpperSaturationLimit=0.9  LowerSaturationLimit=0
  Ki3 : Gain  Gain=110
  Kp3 : Gain  Gain=0.2
  Sum1 : Sum  Inputs=|++
  Out1 : Outport  VectorParamsAs1DForOutWhenUnconnected=off
  wires:
  Integrator3/1 -> Sum1/2
  Ki3/1 -> Integrator3/1
  Kp3/1 -> Sum1/1
  Sum1/1 -> Out1/1
  error/1 -> Kp3/1, Ki3/1

== system Model_DC_MG/Boost -buck Bi-directional converter DC //CD 1 0.65 kW/Primary Control/PID Orig Boost ==
  error : Inport
  Integrator : Integrator  LimitOutput=on  UpperSaturationLimit=0.9  LowerSaturationLimit=0
  Ki : Gain  Gain=3
  Kp : Gain  Gain=0.02
  Sum1 : Sum  Inputs=|++
  Out1 : Outport  VectorParamsAs1DForOutWhenUnconnected=off
  wires:
  Integrator/1 -> Sum1/2
  Sum1/1 -> Out1/1
  Ki/1 -> Integrator/1
  Kp/1 -> Sum1/1
  error/1 -> Ki/1, Kp/1

== system Model_DC_MG/Boost -buck Bi-directional converter DC //CD 1 0.65 kW/Primary Control/PID Orig Buck ==
  error : Inport
  Integrator : Integrator  LimitOutput=on  UpperSaturationLimit=0.9  LowerSaturationLimit=0
  Ki : Gain  Gain=110
  Kp : Gain  Gain=0.02
  Sum1 : Sum  Inputs=|++
  Out1 : Outport  VectorParamsAs1DForOutWhenUnconnected=off
  wires:
  error/1 -> Kp/1, Ki/1
  Kp/1 -> Sum1/1
  Ki/1 -> Integrator/1
  Sum1/1 -> Out1/1
  Integrator/1 -> Sum1/2

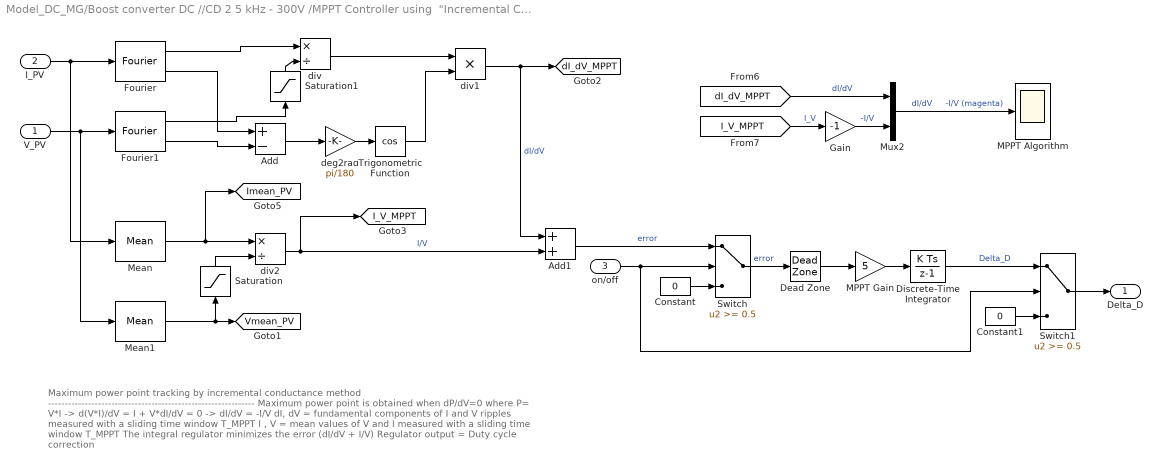
== system Model_DC_MG/Boost converter DC //CD 2 5 kHz - 300V /MPPT Controller using  "Incremental Conductance + Integral Regulator "  technique /MPPT ==
  note: Maximum power point tracking by incremental conductance method
      | --------------------------------------------------------------
      | Maximum power point is obtained when dP/dV=0  where P= V*I
      | -> d(V*I)/dV = I + V*dI/dV = 0
      | -> dI/dV = -I/V
      |
      | dI, dV  = fundamental components of I and V ripples measured with a sliding time window T_MPPT
      | I , V   = mean values of V and I measured with a sliding time window T_MPPT
      |
      | The integral regulator minimizes the error (dI/dV + I/V)
      | Regulator output = Duty cycle correction
  V_PV : Inport
  I_PV : Inport  Port=2
  on/off : Inport  Port=3
  Add : Sum  Inputs=+-
  Add1 : Sum
  Constant : Constant  Value=0
  Constant1 : Constant  Value=0
  Dead Zone : DeadZone  LowerValue=-0.05  UpperValue=0.05
  Discrete-Time Integrator : DiscreteIntegrator  SampleTime=Ts_Control  LimitOutput=on  UpperSaturationLimit=1  LowerSaturationLimit=-1  ICPrevOutput=DiscIntNeverNeededParam  ICPrevScaledInput=DiscIntNeverNeededParam
  Fourier : spsFourierLib/Fourier  Freq=1/T_MPPT  n=1  InInit=[0, 0]  Ts=Ts_Control
  Fourier1 : spsFourierLib/Fourier  Freq=1/T_MPPT  n=1  InInit=[0, 0]  Ts=Ts_Control
  Gain : Gain  Gain=-1
  MPPT Gain : Gain  Gain=5
  MPPT Algorithm : Scope
  Mean : spsMeanLib/Mean  Freq=1/T_MPPT  Vinit=0  Ts=Ts_Control
  Mean1 : spsMeanLib/Mean  Freq=1/T_MPPT  Vinit=0  Ts=Ts_Control
  Mux2 : Mux  Inputs=2
  Saturation : Saturate  UpperLimit=inf  LowerLimit=eps
  Saturation1 : Saturate  UpperLimit=inf  LowerLimit=eps
  Switch : Switch  Threshold=0.5  SaturateOnIntegerOverflow=off  InputSameDT=off
  Switch1 : Switch  Threshold=0.5  SaturateOnIntegerOverflow=off  InputSameDT=off
  Trigonometric Function : Trigonometry  Operator=cos
  deg2rad : Gain  Gain=pi/180
  div : Product  Inputs=*/  RndMeth=Zero
  div1 : Product  Inputs=**  RndMeth=Zero
  div2 : Product  Inputs=*/  RndMeth=Zero
  Delta_D : Outport  VectorParamsAs1DForOutWhenUnconnected=off
  tag scope: I_V_MPPT=global, Imean_PV=global, Vmean_PV=global, dI_dV_MPPT=global
  wires:
  Dead Zone/1 -> MPPT Gain/1
  Switch/1 -> Dead Zone/1  "error"
  Saturation1/1 -> div/2
  Saturation/1 -> div2/2
  Switch1/1 -> Delta_D/1
  on/off/1 -> Switch/2, Switch1/2
  Constant1/1 -> Switch1/3
  Discrete-Time Integrator/1 -> Switch1/1  "Delta_D"
  Constant/1 -> Switch/3
  MPPT Gain/1 -> Discrete-Time Integrator/1
  Add1/1 -> Switch/1  "error"
  div2/1 -> Add1/2, [I_V_MPPT]  "I/V"
  Mean1/1 -> Saturation/1, [Vmean_PV]
  Mean/1 -> div2/1, [Imean_PV]
  div1/1 -> Add1/1, [dI_dV_MPPT]  "dI/dV"
  Trigonometric Function/1 -> div1/2
  div/1 -> div1/1
  deg2rad/1 -> Trigonometric Function/1
  Add/1 -> deg2rad/1
  Fourier1/1 -> Saturation1/1
  Fourier1/2 -> Add/2
  Fourier/2 -> Add/1
  V_PV/1 -> Mean1/1, Fourier1/1
  I_PV/1 -> Mean/1, Fourier/1
  Fourier/1 -> div/1
  [dI_dV_MPPT] -> Mux2/1  "dI/dV"
  Gain/1 -> Mux2/2  "-I/V"
  Mux2/1 -> MPPT Algorithm/1  "dI/dV     -I/V (magenta)"
  [I_V_MPPT] -> Gain/1  "I_V"

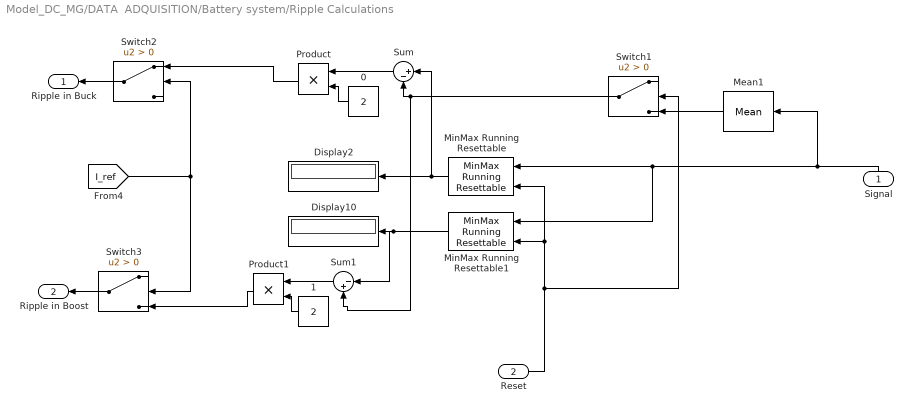
== system Model_DC_MG/DATA  ADQUISITION/Battery system/Ripple Calculations ==
  Signal : Inport
  Reset : Inport  Port=2
  0 : Constant  Value=2
  1 : Constant  Value=2
  Display10 : Display
  Display2 : Display
  Mean1 : spsMeanLib/Mean  Freq=10  Vinit=0  Ts=0
  MinMax Running Resettable : simulink/Math Operations/MinMax Running Resettable  Function=max  vinit=0.0
  MinMax Running Resettable1 : simulink/Math Operations/MinMax Running Resettable  Function=min  vinit=0.0
  Product : Product
  Product1 : Product
  Sum : Sum  Inputs=|+-
  Sum1 : Sum  Inputs=|-+
  Switch1 : Switch  Criteria=u2 > Threshold  SaturateOnIntegerOverflow=off  InputSameDT=off
  Switch2 : Switch  Criteria=u2 > Threshold  SaturateOnIntegerOverflow=off  InputSameDT=off
  Switch3 : Switch  Criteria=u2 > Threshold  SaturateOnIntegerOverflow=off  InputSameDT=off
  Ripple in Buck : Outport  VectorParamsAs1DForOutWhenUnconnected=off
  Ripple in Boost : Outport  Port=2  VectorParamsAs1DForOutWhenUnconnected=off
  wires:
  1/1 -> Product1/2
  [I_ref] -> Switch2/2, Switch3/2
  Product1/1 -> Switch3/3
  0/1 -> Product/2
  Switch2/1 -> Ripple in Buck/1
  Switch3/1 -> Ripple in Boost/1
  Product/1 -> Switch2/1
  Signal/1 -> Mean1/1, MinMax Running Resettable1/1, MinMax Running Resettable/1
  Switch1/1 -> Sum1/2, Sum/2
  MinMax Running Resettable/1 -> Sum/1, Display2/1
  MinMax Running Resettable1/1 -> Sum1/1, Display10/1
  Sum/1 -> Product/1
  Reset/1 -> Switch1/2, MinMax Running Resettable1/2, MinMax Running Resettable/2
  Sum1/1 -> Product1/1
  Mean1/1 -> Switch1/3

== system Model_DC_MG/DATA  ADQUISITION/PV system/Pmean ==
  From7 : From  Commented=on  GotoTag=Vmean_PV
  From8 : From  Commented=on  GotoTag=Imean_PV
  Product : Product  RndMeth=Zero
  WkW : Gain  Gain=1/1000
  P : Outport  VectorParamsAs1DForOutWhenUnconnected=off
  V : Outport  Port=2  VectorParamsAs1DForOutWhenUnconnected=off
  wires:
  [Vdc_bus] -> Product/1, V/1
  Product/1 -> WkW/1
  [I_DC_bus_PV] -> Product/2
  WkW/1 -> P/1  "Pmean_PV (kW)"
